simulink library "gear"  (R2020b)
settings: Solver=VariableStepAuto  StartTime=0.0  StopTime=10.0  RelTol=1e-3
values from neighbouring files (symbols this model uses):
  nge = 0.98    [Projektskript.m]    (also in init.m)
settings Model: Creator=janbantle  LastModifiedBy=Johnathy

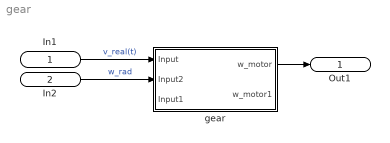
== system gear ==
  In1 : Inport
  In2 : Inport  Port=2
  gear : Subsystem  mask{small_gear=12.5, big_gear=5}
      mask prompts: small_gear "1. Gang"; big_gear "2. Gang"
  Out1 : Outport
  wires:
  In1/1 -> gear/1(Input)  "v_real(t)"
  In2/1 -> gear/2(Input2)  "w_rad"
  gear/1(w_motor) -> Out1/1

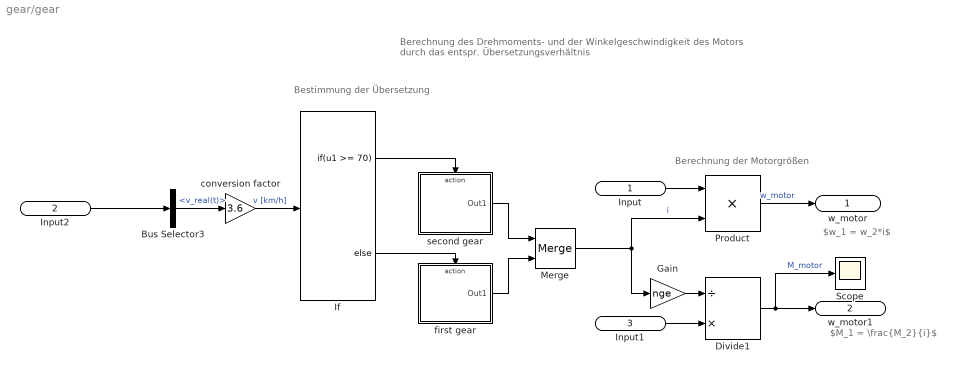
== system gear/gear ==
  note: Berechnung des Drehmoments- und der Winkelgeschwindigkeit des Motors durch das entspr. Übersetzungsverhältnis
  note: Bestimmung der Übersetzung
  note: Berechnung der Motorgrößen
  note: $w_1 = w_2*i$
  note: $M_1 = \frac{M_2}{i}$
  Input : Inport
  Input2 : Inport  Port=2
  Input1 : Inport  Port=3
  Bus Selector3 : BusSelector  OutputSignals=v_real(t)
  Divide1 : Product  Inputs=/*
  Gain : Gain  Gain=nge
  If : If  IfExpression=u1 >= 70
  Merge : Merge
  Product : Product
  Scope : Scope
  conversion factor : Gain  Gain=3.6
  first gear : Subsystem  TreatAsAtomicUnit=on
  second gear : Subsystem  TreatAsAtomicUnit=on
  w_motor : Outport
  w_motor1 : Outport  Port=2
  wires:
  Bus Selector3/1 -> conversion factor/1  "<v_real(t)>"
  Input2/1 -> Bus Selector3/1
  Input/1 -> Product/1
  conversion factor/1 -> If/1  "v [km/h]"
  If/1 -> second gear/Action
  If/2 -> first gear/Action
  Merge/1 -> Gain/1, Product/2  "i"
  second gear/1(Out1) -> Merge/1
  Product/1 -> w_motor/1  "w_motor"
  first gear/1(Out1) -> Merge/2
  Input1/1 -> Divide1/2
  Gain/1 -> Divide1/1
  Divide1/1 -> w_motor1/1, Scope/1  "M_motor"

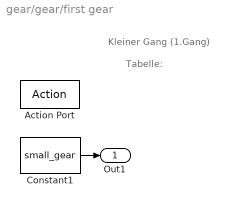
== system gear/gear/first gear ==
  note: Kleiner Gang (1.Gang)
  note: Tabelle:
  Action Port : ActionPort
  Constant1 : Constant  Value=small_gear
  Out1 : Outport
  wires:
  Constant1/1 -> Out1/1

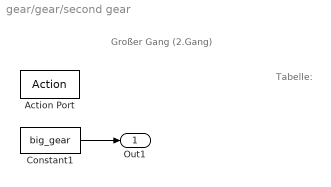
== system gear/gear/second gear ==
  note: Tabelle:
  note: Großer Gang (2.Gang)
  Action Port : ActionPort
  Constant1 : Constant  Value=big_gear
  Out1 : Outport
  wires:
  Constant1/1 -> Out1/1
